simulink model "MLIB_ConvertPU_BAM_F16FLT"  (Simulink 7.3)
settings: Solver=ode45  StartTime=0.0  StopTime=10.0  RelTol=1e-3
settings Model: Creator=RE004C  LastModifiedBy=RE004C
settings HardwareCC: ProdIntDivRoundTo=Zero  ProdEndianess=BigEndian  ProdHWDeviceType=Freescale->32-bit PowerPC

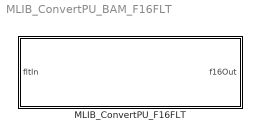
== system MLIB_ConvertPU_BAM_F16FLT ==
  MLIB_ConvertPU_F16FLT : Subsystem  mask(MLIB_ConvertPU_F16){}
      mask help: Bit accurate model for conversion value of input value. Input parameter is considered as single precision floating point value and output value is considered as 16-bit integer value.
      mask init:
      | pos = get_param(gcb, 'Position');width = pos(3) - pos(1); height = pos(4) - pos(2);tX=width/2;tY=height*0.9;
      mask Display: color('black');port_label('input',1,'fltIn');port_label('output',1,'f16Out');color('black');disp('MLIB_ConvertPU_F16FLT');color('blue');text(tX,tY, 'BAM', 'horizontalAlignment', 'center');

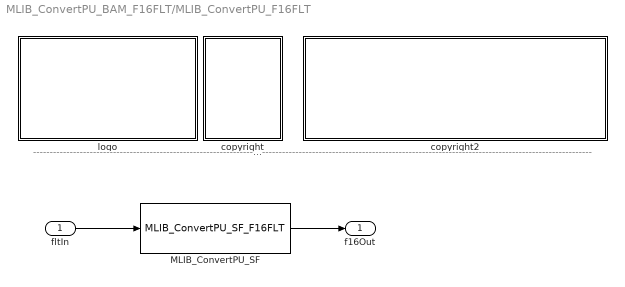
== system MLIB_ConvertPU_BAM_F16FLT/MLIB_ConvertPU_F16FLT ==
  note: ---------------------------------------------------------------------------------------------------------------------------------------------------------------------------------------------------
  fltIn : Inport  OutDataType=fixdt(1, 16)  OutScaling=2^0
  MLIB_ConvertPU_SF : S-Function  FunctionName=MLIB_ConvertPU_SF_F16FLT  EnableBusSupport=off
  copyright : Subsystem
      mask Display: text(10,90,'FILE:');text(10,75,'DESRIPTION:')text(10,60,'COPYRIGHT:')text(10,45,'VERSION:')text(10,30,'DATE:')
  copyright2 : Subsystem
      mask Display: text(10,90,'MLIB_ConvertPU_BAM_F16.mdl');text(10,75,'Converts the input value to different representation in unity model.');text(10,60,'Freescale')text(10,45,'0.1');text(10,30,'10-Oct-2011');
  logo : Subsystem
      mask Display: image(imread('logo.jpg'))
  f16Out : Outport  OutDataType=fixdt(1, 16)  OutScaling=2^0
  wires:
  fltIn/1 -> MLIB_ConvertPU_SF/1
  MLIB_ConvertPU_SF/1 -> f16Out/1

== system MLIB_ConvertPU_BAM_F16FLT/MLIB_ConvertPU_F16FLT/copyright ==

== system MLIB_ConvertPU_BAM_F16FLT/MLIB_ConvertPU_F16FLT/copyright2 ==

== system MLIB_ConvertPU_BAM_F16FLT/MLIB_ConvertPU_F16FLT/logo ==
